simulink model "simulink8"  (R2016b)
settings: Solver=FixedStepAuto  StartTime=0.0  StopTime=30.0  FixedStep=dt  RelTol=1e-3
values from neighbouring files (symbols this model uses):
  A = [   0   0   0   1   0   0 ... (first row only)    [practica8.m]
  B = [   0           0           0           0 ... (first row only)    [practica8.m]
  C = [1  0   0   0   0   0 ... (first row only)    [practica8.m]
  CMD_RATE_LIMIT = 60*pi/180    (= 1.0471975512)    [practica8.m]
  D = zeros(3,4)    [practica8.m]
  K = lqr(A,B,Q,R)    [practica8.m]
  V_bias = 2.0    (= 2)    [practica8.m]
  VMAX_AMP = 24    [practica8.m]
settings Model: Creator=josed  LastModifiedBy=elena
settings DataIOCC: ReturnWorkspaceOutputs=on
settings DebuggingCC: SFMachineParentedDataDiag=error
settings SFSimCC: SimUseLocalCustomCode=on
settings RTWCC: RTWUseLocalCustomCode=on

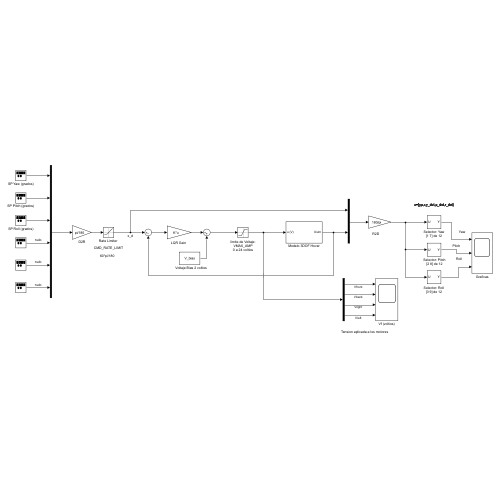
[thumbnail: Simulink's stored preview of the top-level diagram]
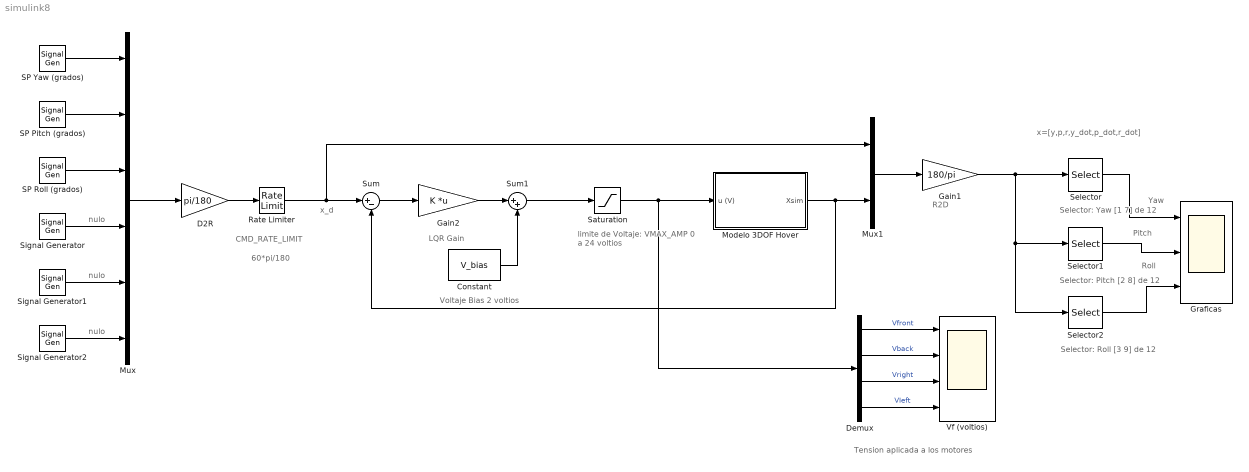
== system simulink8 ==
  note: nulo
  note: x=[y,p,r,y_dot,p_dot,r_dot]
  note: Roll
  note: Pitch
  note: Yaw
  note: Selector: Yaw
      | [1 7] de 12
  note: R2D
  note: Tension aplicada a los motores
  note: limite de Voltaje:
      | VMAX_AMP
      | 0 a 24 voltios
  note: Voltaje Bias 2 voltios
  note: LQR Gain
  note: x_d
  note: 60*pi/180
  note: CMD_RATE_LIMIT
  note: Selector: Pitch
      | [2 8] de 12
  note: Selector: Roll
      | [3 9] de 12
  note: nulo
  note: nulo
  Constant : Constant  Value=V_bias
  D2R : Gain  Gain=pi/180
  Demux : Demux
  Gain1 : Gain  Gain=180/pi
  Gain2 : Gain  Gain=K  Multiplication=Matrix(K*u)
  Graficas : Scope  NumInputPorts=3
  Modelo 3DOF Hover : Subsystem
  Mux : Mux  Inputs=6
  Mux1 : Mux  Inputs=2
  "Rate Limiter " : RateLimiter  RisingSlewLimit=CMD_RATE_LIMIT  FallingSlewLimit=-CMD_RATE_LIMIT  InitialCondition=60*pi/180
  SP Pitch (grados) : SignalGenerator  WaveForm=square  Amplitude=4  Frequency=0.1
  SP Roll (grados) : SignalGenerator  WaveForm=square  Amplitude=4  Frequency=0.08
  SP Yaw (grados) : SignalGenerator  WaveForm=square  Amplitude=5  Frequency=0.04
  Saturation : Saturate  UpperLimit=VMAX_AMP  LowerLimit=0
  Selector : Selector  InputPortWidth=12  IndexOptions=Index vector (dialog)  Indices=[1 7]  OutputSizes=1
  Selector1 : Selector  InputPortWidth=12  IndexOptions=Index vector (dialog)  Indices=[2 8]  OutputSizes=1
  Selector2 : Selector  InputPortWidth=12  IndexOptions=Index vector (dialog)  Indices=[3 9]  OutputSizes=1
  Signal Generator : SignalGenerator  WaveForm=square  Amplitude=0  Frequency=0.1
  Signal Generator1 : SignalGenerator  WaveForm=square  Amplitude=0  Frequency=0.1
  Signal Generator2 : SignalGenerator  WaveForm=square  Amplitude=0  Frequency=0.1
  Sum : Sum  Inputs=|+-
  Sum1 : Sum  Inputs=|++
  Vf (voltios) : Scope  NumInputPorts=4
  wires:
  SP Yaw (grados)/1 -> Mux/1
  SP Pitch (grados)/1 -> Mux/2
  SP Roll (grados)/1 -> Mux/3
  Signal Generator/1 -> Mux/4
  Signal Generator1/1 -> Mux/5
  Signal Generator2/1 -> Mux/6
  Mux/1 -> D2R/1
  D2R/1 -> "Rate Limiter "/1
  "Rate Limiter "/1 -> Mux1/1, Sum/1
  Sum1/1 -> Saturation/1
  Gain2/1 -> Sum1/1
  Sum/1 -> Gain2/1
  Constant/1 -> Sum1/2
  Saturation/1 -> Demux/1, Modelo 3DOF Hover/1(u (V))
  Modelo 3DOF Hover/1(Xsim) -> Sum/2, Mux1/2
  Demux/1 -> Vf (voltios)/1  "Vfront"
  Demux/2 -> Vf (voltios)/2  "Vback"
  Demux/3 -> Vf (voltios)/3  "Vright"
  Demux/4 -> Vf (voltios)/4  "VIeft"
  Mux1/1 -> Gain1/1
  Gain1/1 -> Selector1/1, Selector2/1, Selector/1
  Selector/1 -> Graficas/1
  Selector1/1 -> Graficas/2
  Selector2/1 -> Graficas/3

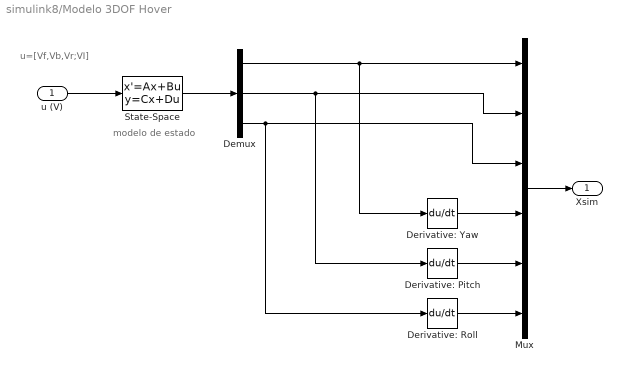
== system simulink8/Modelo 3DOF Hover ==
  note: modelo de estado
  note: u=[Vf,Vb,Vr;VI]
  u (V) : Inport
  Demux : Demux  Outputs=3
  Derivative: Pitch : Derivative
  Derivative: Roll : Derivative
  Derivative: Yaw : Derivative
  Mux : Mux  Inputs=6
  State-Space : StateSpace  A=A  B=B  C=C  D=D  X0=0
  Xsim : Outport
  wires:
  State-Space/1 -> Demux/1
  u (V)/1 -> State-Space/1
  Demux/1 -> Derivative: Yaw/1, Mux/1
  Demux/2 -> Derivative: Pitch/1, Mux/2
  Demux/3 -> Derivative: Roll/1, Mux/3
  Derivative: Yaw/1 -> Mux/4
  Derivative: Pitch/1 -> Mux/5
  Derivative: Roll/1 -> Mux/6
  Mux/1 -> Xsim/1
